simulink model "GalacticSoupLogical"  (R2025b)
settings: Solver=VariableStepAuto  StartTime=0.0  StopTime=10.0  RelTol=1e-3
settings Model: DataDictionary=GalacticSoupLogicalInterfaces.sldd  Creator=sarah  LastModifiedBy=sarah

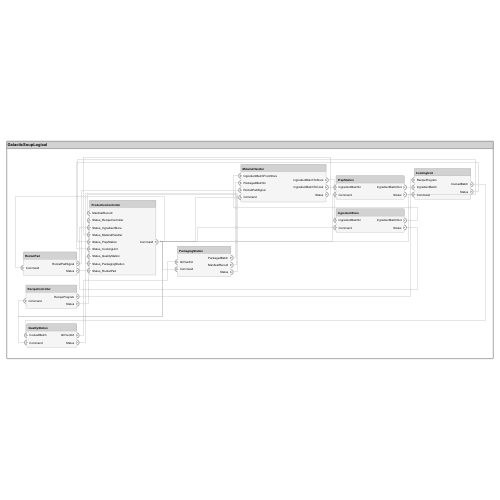
[thumbnail: Simulink's stored preview of the top-level diagram]
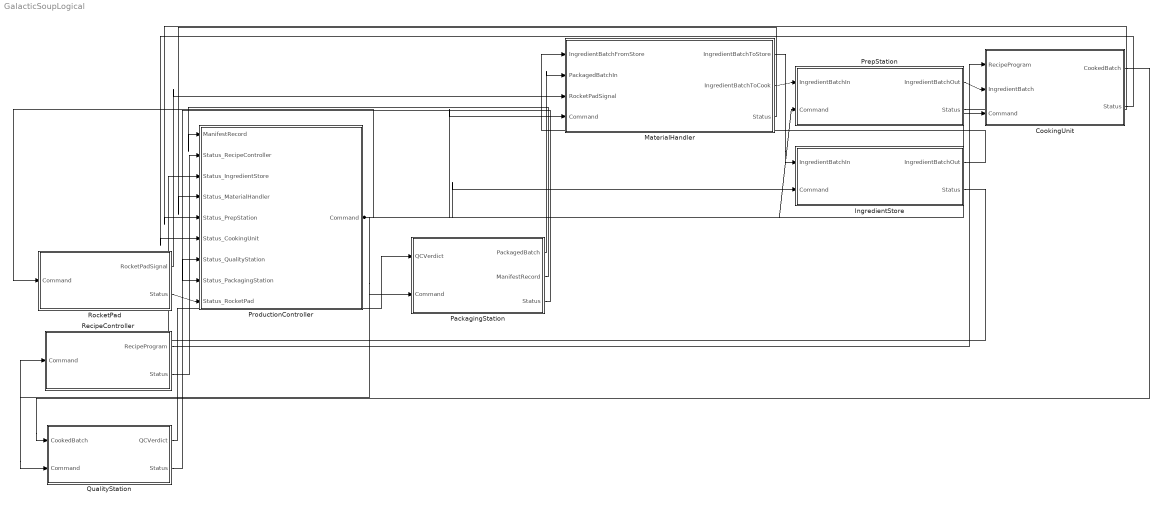
== system GalacticSoupLogical ==
  CookingUnit : Subsystem
      settings: PortSchema="{\"entries\":[{\"content\":{\"headerSize\":26,\"margin\":15,\"minimumSpacing\":25,\"sides\":[{\"content\":{\"connectorIds\":[\"In1\",\"In2\",\"In3\"]},\"type\":\"ConnectorPlacement.EquallySpacedRectSide\",\"uuid\":\"47548036-a6c3-440f-b573-2a4e753e82ae\"},{\"content\":{\"connectorIds\":[\"Out1\",\"Out2\"],\"side\":\"RIGHT\"},\"type\":\"ConnectorPlacement.EquallySpacedRectSide\",\"uuid\":\"ab096620-2054-4429-8520-52cfe6541bb8\"},{\"content\":{\"side\":\"TOP\"},\"type\":\"ConnectorPlacement.EquallySpacedRectSide\",\"uuid\":\"6e18e29c-ba68-48ca-8847-f496b38e15b5\"}]},\"type\":\"ConnectorPlacement.EquallySpacedConnector\",\"uuid\":\"7233fc04-a641-40d9-8870-909b934a9733\"}],\"packageUris\":[\"http://schema.mathworks.com/mf0/Connector/R2020b\"],\"version\":\"1.0\"}"
  IngredientStore : Subsystem
      settings: PortSchema="{\"entries\":[{\"content\":{\"headerSize\":26,\"margin\":15,\"minimumSpacing\":25,\"sides\":[{\"content\":{\"connectorIds\":[\"In1\",\"In2\"]},\"type\":\"ConnectorPlacement.EquallySpacedRectSide\",\"uuid\":\"47548036-a6c3-440f-b573-2a4e753e82ae\"},{\"content\":{\"connectorIds\":[\"Out1\",\"Out2\"],\"side\":\"RIGHT\"},\"type\":\"ConnectorPlacement.EquallySpacedRectSide\",\"uuid\":\"ab096620-2054-4429-8520-52cfe6541bb8\"},{\"content\":{\"side\":\"TOP\"},\"type\":\"ConnectorPlacement.EquallySpacedRectSide\",\"uuid\":\"6e18e29c-ba68-48ca-8847-f496b38e15b5\"}]},\"type\":\"ConnectorPlacement.EquallySpacedConnector\",\"uuid\":\"7233fc04-a641-40d9-8870-909b934a9733\"}],\"packageUris\":[\"http://schema.mathworks.com/mf0/Connector/R2020b\"],\"version\":\"1.0\"}"
  MaterialHandler : Subsystem
      settings: PortSchema="{\"entries\":[{\"content\":{\"headerSize\":26,\"margin\":15,\"minimumSpacing\":25,\"sides\":[{\"content\":{\"connectorIds\":[\"In1\",\"In2\",\"In3\",\"In4\"]},\"type\":\"ConnectorPlacement.EquallySpacedRectSide\",\"uuid\":\"47548036-a6c3-440f-b573-2a4e753e82ae\"},{\"content\":{\"connectorIds\":[\"Out1\",\"Out2\",\"Out3\"],\"side\":\"RIGHT\"},\"type\":\"ConnectorPlacement.EquallySpacedRectSide\",\"uuid\":\"ab096620-2054-4429-8520-52cfe6541bb8\"},{\"content\":{\"side\":\"TOP\"},\"type\":\"ConnectorPlacement.EquallySpacedRectSide\",\"uuid\":\"6e18e29c-ba68-48ca-8847-f496b38e15b5\"}]},\"type\":\"ConnectorPlacement.EquallySpacedConnector\",\"uuid\":\"7233fc04-a641-40d9-8870-909b934a9733\"}],\"packageUris\":[\"http://schema.mathworks.com/mf0/Connector/R2020b\"],\"version\":\"1.0\"}"
  PackagingStation : Subsystem
      settings: PortSchema="{\"entries\":[{\"content\":{\"headerSize\":26,\"margin\":15,\"minimumSpacing\":25,\"sides\":[{\"content\":{\"connectorIds\":[\"In1\",\"In2\"]},\"type\":\"ConnectorPlacement.EquallySpacedRectSide\",\"uuid\":\"47548036-a6c3-440f-b573-2a4e753e82ae\"},{\"content\":{\"connectorIds\":[\"Out1\",\"Out2\",\"Out3\"],\"side\":\"RIGHT\"},\"type\":\"ConnectorPlacement.EquallySpacedRectSide\",\"uuid\":\"ab096620-2054-4429-8520-52cfe6541bb8\"},{\"content\":{\"side\":\"TOP\"},\"type\":\"ConnectorPlacement.EquallySpacedRectSide\",\"uuid\":\"6e18e29c-ba68-48ca-8847-f496b38e15b5\"}]},\"type\":\"ConnectorPlacement.EquallySpacedConnector\",\"uuid\":\"7233fc04-a641-40d9-8870-909b934a9733\"}],\"packageUris\":[\"http://schema.mathworks.com/mf0/Connector/R2020b\"],\"version\":\"1.0\"}"
  PrepStation : Subsystem
      settings: PortSchema="{\"entries\":[{\"content\":{\"headerSize\":26,\"margin\":15,\"minimumSpacing\":25,\"sides\":[{\"content\":{\"connectorIds\":[\"In1\",\"In2\"]},\"type\":\"ConnectorPlacement.EquallySpacedRectSide\",\"uuid\":\"47548036-a6c3-440f-b573-2a4e753e82ae\"},{\"content\":{\"connectorIds\":[\"Out1\",\"Out2\"],\"side\":\"RIGHT\"},\"type\":\"ConnectorPlacement.EquallySpacedRectSide\",\"uuid\":\"ab096620-2054-4429-8520-52cfe6541bb8\"},{\"content\":{\"side\":\"TOP\"},\"type\":\"ConnectorPlacement.EquallySpacedRectSide\",\"uuid\":\"6e18e29c-ba68-48ca-8847-f496b38e15b5\"}]},\"type\":\"ConnectorPlacement.EquallySpacedConnector\",\"uuid\":\"7233fc04-a641-40d9-8870-909b934a9733\"}],\"packageUris\":[\"http://schema.mathworks.com/mf0/Connector/R2020b\"],\"version\":\"1.0\"}"
  ProductionController : Subsystem
      settings: PortSchema="{\"entries\":[{\"content\":{\"headerSize\":26,\"margin\":15,\"minimumSpacing\":25,\"sides\":[{\"content\":{\"connectorIds\":[\"In1\",\"In2\",\"In3\",\"In4\",\"In5\",\"In6\",\"In7\",\"In8\",\"In9\"]},\"type\":\"ConnectorPlacement.EquallySpacedRectSide\",\"uuid\":\"47548036-a6c3-440f-b573-2a4e753e82ae\"},{\"content\":{\"connectorIds\":[\"Out1\"],\"side\":\"RIGHT\"},\"type\":\"ConnectorPlacement.EquallySpacedRectSide\",\"uuid\":\"ab096620-2054-4429-8520-52cfe6541bb8\"},{\"content\":{\"side\":\"TOP\"},\"type\":\"ConnectorPlacement.EquallySpacedRectSide\",\"uuid\":\"6e18e29c-ba68-48ca-8847-f496b38e15b5\"}]},\"type\":\"ConnectorPlacement.EquallySpacedConnector\",\"uuid\":\"7233fc04-a641-40d9-8870-909b934a9733\"}],\"packageUris\":[\"http://schema.mathworks.com/mf0/Connector/R2020b\"],\"version\":\"1.0\"}"
  QualityStation : Subsystem
      settings: PortSchema="{\"entries\":[{\"content\":{\"headerSize\":26,\"margin\":15,\"minimumSpacing\":25,\"sides\":[{\"content\":{\"connectorIds\":[\"In1\",\"In2\"]},\"type\":\"ConnectorPlacement.EquallySpacedRectSide\",\"uuid\":\"47548036-a6c3-440f-b573-2a4e753e82ae\"},{\"content\":{\"connectorIds\":[\"Out1\",\"Out2\"],\"side\":\"RIGHT\"},\"type\":\"ConnectorPlacement.EquallySpacedRectSide\",\"uuid\":\"ab096620-2054-4429-8520-52cfe6541bb8\"},{\"content\":{\"side\":\"TOP\"},\"type\":\"ConnectorPlacement.EquallySpacedRectSide\",\"uuid\":\"6e18e29c-ba68-48ca-8847-f496b38e15b5\"}]},\"type\":\"ConnectorPlacement.EquallySpacedConnector\",\"uuid\":\"7233fc04-a641-40d9-8870-909b934a9733\"}],\"packageUris\":[\"http://schema.mathworks.com/mf0/Connector/R2020b\"],\"version\":\"1.0\"}"
  RecipeController : Subsystem
      settings: PortSchema="{\"entries\":[{\"content\":{\"headerSize\":26,\"margin\":15,\"minimumSpacing\":25,\"sides\":[{\"content\":{\"connectorIds\":[\"In1\"]},\"type\":\"ConnectorPlacement.EquallySpacedRectSide\",\"uuid\":\"47548036-a6c3-440f-b573-2a4e753e82ae\"},{\"content\":{\"connectorIds\":[\"Out1\",\"Out2\"],\"side\":\"RIGHT\"},\"type\":\"ConnectorPlacement.EquallySpacedRectSide\",\"uuid\":\"ab096620-2054-4429-8520-52cfe6541bb8\"},{\"content\":{\"side\":\"TOP\"},\"type\":\"ConnectorPlacement.EquallySpacedRectSide\",\"uuid\":\"6e18e29c-ba68-48ca-8847-f496b38e15b5\"}]},\"type\":\"ConnectorPlacement.EquallySpacedConnector\",\"uuid\":\"7233fc04-a641-40d9-8870-909b934a9733\"}],\"packageUris\":[\"http://schema.mathworks.com/mf0/Connector/R2020b\"],\"version\":\"1.0\"}"
  RocketPad : Subsystem
      settings: PortSchema="{\"entries\":[{\"content\":{\"headerSize\":26,\"margin\":15,\"minimumSpacing\":25,\"sides\":[{\"content\":{\"connectorIds\":[\"In1\"]},\"type\":\"ConnectorPlacement.EquallySpacedRectSide\",\"uuid\":\"47548036-a6c3-440f-b573-2a4e753e82ae\"},{\"content\":{\"connectorIds\":[\"Out1\",\"Out2\"],\"side\":\"RIGHT\"},\"type\":\"ConnectorPlacement.EquallySpacedRectSide\",\"uuid\":\"ab096620-2054-4429-8520-52cfe6541bb8\"},{\"content\":{\"side\":\"TOP\"},\"type\":\"ConnectorPlacement.EquallySpacedRectSide\",\"uuid\":\"6e18e29c-ba68-48ca-8847-f496b38e15b5\"}]},\"type\":\"ConnectorPlacement.EquallySpacedConnector\",\"uuid\":\"7233fc04-a641-40d9-8870-909b934a9733\"}],\"packageUris\":[\"http://schema.mathworks.com/mf0/Connector/R2020b\"],\"version\":\"1.0\"}"
  wires:
  QualityStation/2(Status) -> ProductionController/7(Status_QualityStation)
  RocketPad/1(RocketPadSignal) -> MaterialHandler/3(RocketPadSignal)
  ProductionController/1(Command) -> RecipeController/1(Command), QualityStation/2(Command), PrepStation/2(Command), MaterialHandler/4(Command), CookingUnit/3(Command), IngredientStore/2(Command), RocketPad/1(Command), PackagingStation/2(Command)
  RecipeController/2(Status) -> ProductionController/2(Status_RecipeController)
  IngredientStore/2(Status) -> ProductionController/3(Status_IngredientStore)
  RocketPad/2(Status) -> ProductionController/9(Status_RocketPad)
  RecipeController/1(RecipeProgram) -> CookingUnit/1(RecipeProgram)
  QualityStation/1(QCVerdict) -> PackagingStation/1(QCVerdict)
  PackagingStation/1(PackagedBatch) -> MaterialHandler/2(PackagedBatchIn)
  PackagingStation/2(ManifestRecord) -> ProductionController/1(ManifestRecord)
  PackagingStation/3(Status) -> ProductionController/8(Status_PackagingStation)
  MaterialHandler/1(IngredientBatchToStore) -> IngredientStore/1(IngredientBatchIn)
  MaterialHandler/2(IngredientBatchToCook) -> PrepStation/1(IngredientBatchIn)
  MaterialHandler/3(Status) -> ProductionController/4(Status_MaterialHandler)
  PrepStation/1(IngredientBatchOut) -> CookingUnit/2(IngredientBatch)
  PrepStation/2(Status) -> ProductionController/5(Status_PrepStation)
  IngredientStore/1(IngredientBatchOut) -> MaterialHandler/1(IngredientBatchFromStore)
  CookingUnit/1(CookedBatch) -> QualityStation/1(CookedBatch)
  CookingUnit/2(Status) -> ProductionController/6(Status_CookingUnit)

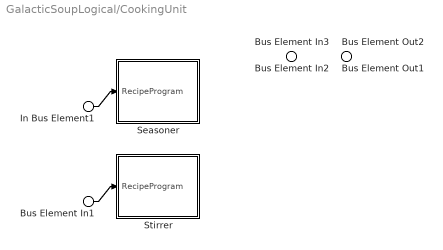
== system GalacticSoupLogical/CookingUnit ==
  Bus Element In1 : Inport  PortName=RecipeProgram
  In Bus Element1 : Inport  PortName=RecipeProgram
  Bus Element In2 : Inport  Port=2  PortName=IngredientBatch
  Bus Element In3 : Inport  Port=3  PortName=Command
  Seasoner : Subsystem
      settings: PortSchema="{\"entries\":[{\"content\":{\"headerSize\":26,\"margin\":15,\"minimumSpacing\":25,\"sides\":[{\"content\":{\"connectorIds\":[\"In1\"]},\"type\":\"ConnectorPlacement.EquallySpacedRectSide\",\"uuid\":\"47548036-a6c3-440f-b573-2a4e753e82ae\"},{\"content\":{\"side\":\"RIGHT\"},\"type\":\"ConnectorPlacement.EquallySpacedRectSide\",\"uuid\":\"ab096620-2054-4429-8520-52cfe6541bb8\"},{\"content\":{\"side\":\"TOP\"},\"type\":\"ConnectorPlacement.EquallySpacedRectSide\",\"uuid\":\"6e18e29c-ba68-48ca-8847-f496b38e15b5\"}]},\"type\":\"ConnectorPlacement.EquallySpacedConnector\",\"uuid\":\"7233fc04-a641-40d9-8870-909b934a9733\"}],\"packageUris\":[\"http://schema.mathworks.com/mf0/Connector/R2020b\"],\"version\":\"1.0\"}"
  Stirrer : Subsystem
      settings: PortSchema="{\"entries\":[{\"content\":{\"headerSize\":26,\"margin\":15,\"minimumSpacing\":25,\"sides\":[{\"content\":{\"connectorIds\":[\"In1\"]},\"type\":\"ConnectorPlacement.EquallySpacedRectSide\",\"uuid\":\"47548036-a6c3-440f-b573-2a4e753e82ae\"},{\"content\":{\"side\":\"RIGHT\"},\"type\":\"ConnectorPlacement.EquallySpacedRectSide\",\"uuid\":\"ab096620-2054-4429-8520-52cfe6541bb8\"},{\"content\":{\"side\":\"TOP\"},\"type\":\"ConnectorPlacement.EquallySpacedRectSide\",\"uuid\":\"6e18e29c-ba68-48ca-8847-f496b38e15b5\"}]},\"type\":\"ConnectorPlacement.EquallySpacedConnector\",\"uuid\":\"7233fc04-a641-40d9-8870-909b934a9733\"}],\"packageUris\":[\"http://schema.mathworks.com/mf0/Connector/R2020b\"],\"version\":\"1.0\"}"
  Bus Element Out1 : Outport  PortName=CookedBatch
  Bus Element Out2 : Outport  Port=2  PortName=Status
  wires:
  In Bus Element1/1 -> Seasoner/1(RecipeProgram)
  Bus Element In1/1 -> Stirrer/1(RecipeProgram)

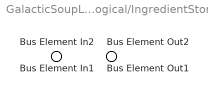
== system GalacticSoupLogical/IngredientStore ==
  Bus Element In1 : Inport  PortName=IngredientBatchIn
  Bus Element In2 : Inport  Port=2  PortName=Command
  Bus Element Out1 : Outport  PortName=IngredientBatchOut
  Bus Element Out2 : Outport  Port=2  PortName=Status

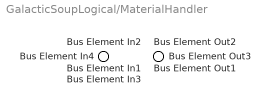
== system GalacticSoupLogical/MaterialHandler ==
  Bus Element In1 : Inport  PortName=IngredientBatchFromStore
  Bus Element In2 : Inport  Port=2  PortName=PackagedBatchIn
  Bus Element In3 : Inport  Port=3  PortName=RocketPadSignal
  Bus Element In4 : Inport  Port=4  PortName=Command
  Bus Element Out1 : Outport  PortName=IngredientBatchToStore
  Bus Element Out2 : Outport  Port=2  PortName=IngredientBatchToCook
  Bus Element Out3 : Outport  Port=3  PortName=Status

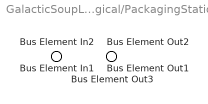
== system GalacticSoupLogical/PackagingStation ==
  Bus Element In1 : Inport  PortName=QCVerdict
  Bus Element In2 : Inport  Port=2  PortName=Command
  Bus Element Out1 : Outport  PortName=PackagedBatch
  Bus Element Out2 : Outport  Port=2  PortName=ManifestRecord
  Bus Element Out3 : Outport  Port=3  PortName=Status

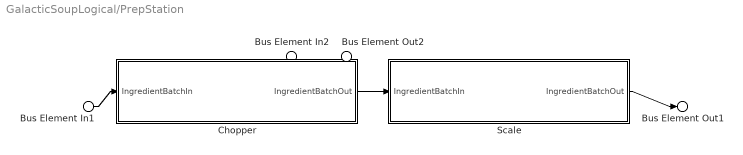
== system GalacticSoupLogical/PrepStation ==
  Bus Element In1 : Inport  PortName=IngredientBatchIn
  Bus Element In2 : Inport  Port=2  PortName=Command
  Chopper : Subsystem
      settings: PortSchema="{\"entries\":[{\"content\":{\"headerSize\":26,\"margin\":15,\"minimumSpacing\":25,\"sides\":[{\"content\":{\"connectorIds\":[\"In1\"]},\"type\":\"ConnectorPlacement.EquallySpacedRectSide\",\"uuid\":\"47548036-a6c3-440f-b573-2a4e753e82ae\"},{\"content\":{\"connectorIds\":[\"Out1\"],\"side\":\"RIGHT\"},\"type\":\"ConnectorPlacement.EquallySpacedRectSide\",\"uuid\":\"ab096620-2054-4429-8520-52cfe6541bb8\"},{\"content\":{\"side\":\"TOP\"},\"type\":\"ConnectorPlacement.EquallySpacedRectSide\",\"uuid\":\"6e18e29c-ba68-48ca-8847-f496b38e15b5\"}]},\"type\":\"ConnectorPlacement.EquallySpacedConnector\",\"uuid\":\"7233fc04-a641-40d9-8870-909b934a9733\"}],\"packageUris\":[\"http://schema.mathworks.com/mf0/Connector/R2020b\"],\"version\":\"1.0\"}"
  Scale : Subsystem
      settings: PortSchema="{\"entries\":[{\"content\":{\"headerSize\":26,\"margin\":15,\"minimumSpacing\":25,\"sides\":[{\"content\":{\"connectorIds\":[\"In1\"]},\"type\":\"ConnectorPlacement.EquallySpacedRectSide\",\"uuid\":\"47548036-a6c3-440f-b573-2a4e753e82ae\"},{\"content\":{\"connectorIds\":[\"Out1\"],\"side\":\"RIGHT\"},\"type\":\"ConnectorPlacement.EquallySpacedRectSide\",\"uuid\":\"ab096620-2054-4429-8520-52cfe6541bb8\"},{\"content\":{\"side\":\"TOP\"},\"type\":\"ConnectorPlacement.EquallySpacedRectSide\",\"uuid\":\"6e18e29c-ba68-48ca-8847-f496b38e15b5\"}]},\"type\":\"ConnectorPlacement.EquallySpacedConnector\",\"uuid\":\"7233fc04-a641-40d9-8870-909b934a9733\"}],\"packageUris\":[\"http://schema.mathworks.com/mf0/Connector/R2020b\"],\"version\":\"1.0\"}"
  Bus Element Out1 : Outport  PortName=IngredientBatchOut
  Bus Element Out2 : Outport  Port=2  PortName=Status
  wires:
  Bus Element In1/1 -> Chopper/1(IngredientBatchIn)
  Chopper/1(IngredientBatchOut) -> Scale/1(IngredientBatchIn)
  Scale/1(IngredientBatchOut) -> Bus Element Out1/1

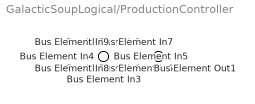
== system GalacticSoupLogical/ProductionController ==
  Bus Element In1 : Inport  PortName=ManifestRecord
  Bus Element In2 : Inport  Port=2  PortName=Status_RecipeController
  Bus Element In3 : Inport  Port=3  PortName=Status_IngredientStore
  Bus Element In4 : Inport  Port=4  PortName=Status_MaterialHandler
  Bus Element In5 : Inport  Port=5  PortName=Status_PrepStation
  Bus Element In6 : Inport  Port=6  PortName=Status_CookingUnit
  Bus Element In7 : Inport  Port=7  PortName=Status_QualityStation
  Bus Element In8 : Inport  Port=8  PortName=Status_PackagingStation
  Bus Element In9 : Inport  Port=9  PortName=Status_RocketPad
  Bus Element Out1 : Outport  PortName=Command

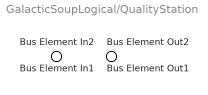
== system GalacticSoupLogical/QualityStation ==
  Bus Element In1 : Inport  PortName=CookedBatch
  Bus Element In2 : Inport  Port=2  PortName=Command
  Bus Element Out1 : Outport  PortName=QCVerdict
  Bus Element Out2 : Outport  Port=2  PortName=Status

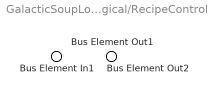
== system GalacticSoupLogical/RecipeController ==
  Bus Element In1 : Inport  PortName=Command
  Bus Element Out1 : Outport  PortName=RecipeProgram
  Bus Element Out2 : Outport  Port=2  PortName=Status

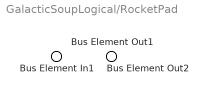
== system GalacticSoupLogical/RocketPad ==
  Bus Element In1 : Inport  PortName=Command
  Bus Element Out1 : Outport  PortName=RocketPadSignal
  Bus Element Out2 : Outport  Port=2  PortName=Status

== system GalacticSoupLogical/CookingUnit/Seasoner ==
  Bus Element In1 : Inport  PortName=RecipeProgram

== system GalacticSoupLogical/CookingUnit/Stirrer ==
  Bus Element In1 : Inport  PortName=RecipeProgram

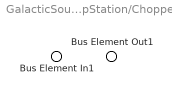
== system GalacticSoupLogical/PrepStation/Chopper ==
  Bus Element In1 : Inport  PortName=IngredientBatchIn
  Bus Element Out1 : Outport  PortName=IngredientBatchOut

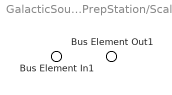
== system GalacticSoupLogical/PrepStation/Scale ==
  Bus Element In1 : Inport  PortName=IngredientBatchIn
  Bus Element Out1 : Outport  PortName=IngredientBatchOut
